simulink model "sl_subsys_trigerr1"  (Simulink 6.0)
settings: Solver=ode45  StartTime=0.0  StopTime=10.0  RelTol=1e-3
settings Model: CovMetricSettings=d  Creator=The MathWorks Inc.  LastModifiedBy=batserve  ExtModeAutoUpdateStatusClock=off
settings OptimizationCC: BlockReduction=off  BooleanDataType=off
settings DebuggingCC: CheckExecutionContextPreStartOutputMsg=on  CheckExecutionContextRuntimeOutputMsg=on  SolverPrmCheckMsg=none
settings HardwareCC: TargetUnknown=on

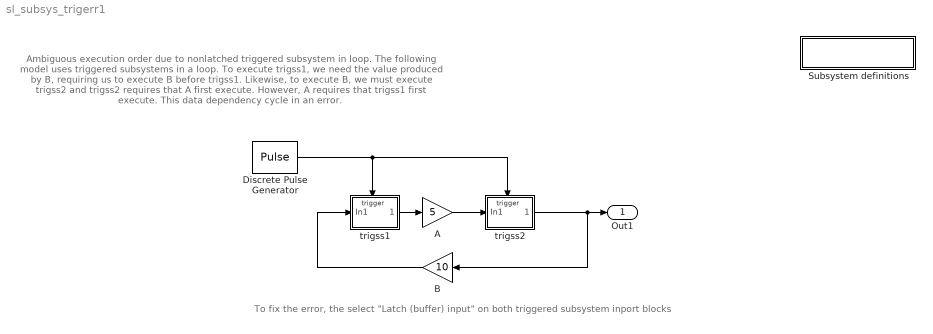
== system sl_subsys_trigerr1 ==
  note: Ambiguous execution order due to nonlatched triggered subsystem in loop.
      |
      | The following model uses triggered subsystems in a loop. To execute
      | trigss1, we need the value produced by B, requiring us to execute
      | B before trigss1. Likewise, to execute B, we must execute trigss2
      | and trigss2 requires that A first execute. However, A requires that
      | trigss1 first execute. This data dependency cycle in an error.
  note: To fix the error, the select "Latch (buffer) input" on both triggered subsystem inport blocks
  " Subsystem definitions" : Subsystem  PropExecContextAcrossSSBoundary=on
      settings: OpenFcn=helpview([matlabroot,'/toolbox/simulink/simdemos/sl_subsys_definitions.html']);
      mask Display: disp('Subsystem\ndefinitions')
  A : Gain  Gain=5  SaturateOnIntegerOverflow=on
  B : Gain  Orientation=left  Gain=10  SaturateOnIntegerOverflow=on
  Discrete Pulse Generator : DiscretePulseGenerator
  trigss1 : Subsystem  TreatAsAtomicUnit=on  PropExecContextAcrossSSBoundary=on
  trigss2 : Subsystem  TreatAsAtomicUnit=on  PropExecContextAcrossSSBoundary=on
  Out1 : Outport
  wires:
  trigss1/1(Out1) -> A/1
  A/1 -> trigss2/1(In1)
  trigss2/1(Out1) -> B/1, Out1/1
  B/1 -> trigss1/1(In1)
  Discrete Pulse Generator/1 -> trigss1/Trigger, trigss2/Trigger

== system sl_subsys_trigerr1/ Subsystem definitions ==

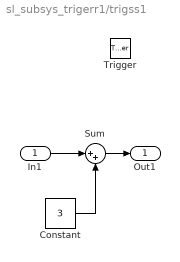
== system sl_subsys_trigerr1/trigss1 ==
  In1 : Inport  Port=1  LatchInput=off
  Trigger : TriggerPort
  Constant : Constant  Value=3
  Sum : Sum  Inputs=|++  SaturateOnIntegerOverflow=on  InputSameDT=on
  Out1 : Outport
  wires:
  In1/1 -> Sum/1
  Sum/1 -> Out1/1
  Constant/1 -> Sum/2

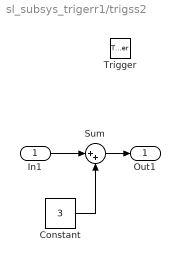
== system sl_subsys_trigerr1/trigss2 ==
  In1 : Inport  Port=1  LatchInput=off
  Trigger : TriggerPort
  Constant : Constant  Value=3
  Sum : Sum  Inputs=|++  SaturateOnIntegerOverflow=on  InputSameDT=on
  Out1 : Outport
  wires:
  Constant/1 -> Sum/2
  Sum/1 -> Out1/1
  In1/1 -> Sum/1
